simulink model "sim3_3"  (R2019a)
settings: Solver=VariableStepAuto  StartTime=0.0  StopTime=10.0  RelTol=1e-3
values from neighbouring files (symbols this model uses):
  h = 0.2    [matlab3_3.m]
  Ki_a = 25    [matlab3_3.m]
  Ki_d = Ki_a * h / 2    (= 2.5)    [matlab3_3.m]
  Kp_a = 6    [matlab3_3.m]
  Kp_d = Kp_a    (= 6)    [matlab3_3.m]
undefined symbols (not defined in the file or in its folder): denG, numG
settings Model: Creator=User  LastModifiedBy=User

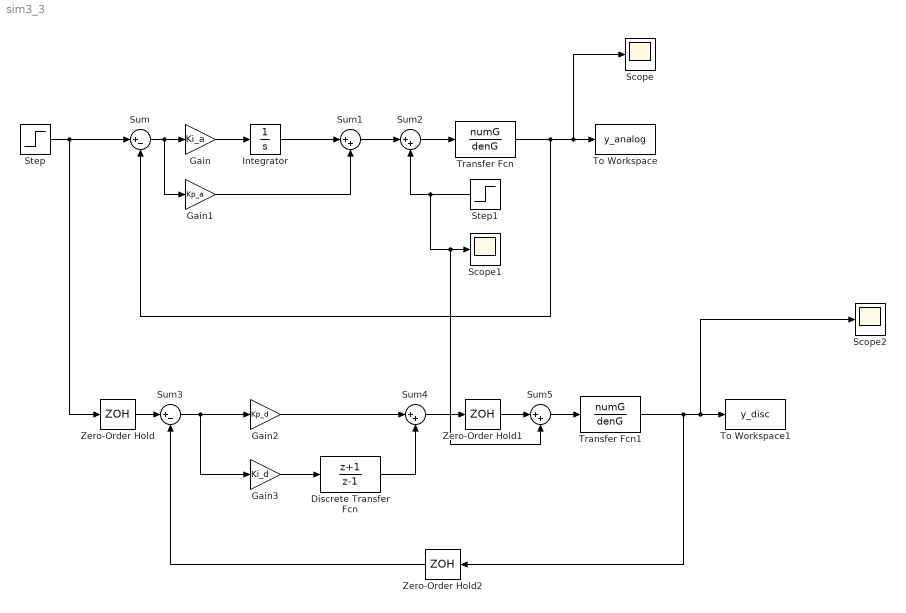
== system sim3_3 ==
  Discrete Transfer Fcn : DiscreteTransferFcn  Numerator=[1 1]  Denominator=[1 -1]  SampleTime=h
  Gain : Gain  Gain=Ki_a
  Gain1 : Gain  Gain=Kp_a
  Gain2 : Gain  Gain=Kp_d
  Gain3 : Gain  Gain=Ki_d
  Integrator : Integrator
  Scope : Scope
  Scope1 : Scope
  Scope2 : Scope
  Step : Step  SampleTime=0
  Step1 : Step  Time=0  After=0  SampleTime=0
  Sum : Sum  Inputs=|+-
  Sum{1..2,4..5} (4 alike) : Sum  Inputs=|++
  Sum3 : Sum  Inputs=|+-
  To Workspace : ToWorkspace  VariableName=y_analog  SaveFormat=Structure With Time  SampleTime=-1
  To Workspace1 : ToWorkspace  VariableName=y_disc  SaveFormat=Structure With Time  SampleTime=-1
  Transfer Fcn : TransferFcn  Numerator=numG  Denominator=denG
  Transfer Fcn1 : TransferFcn  Numerator=numG  Denominator=denG
  Zero-Order Hold : ZeroOrderHold  SampleTime=h
  Zero-Order Hold1 : ZeroOrderHold  SampleTime=h
  Zero-Order Hold2 : ZeroOrderHold  SampleTime=h
  wires:
  Sum/1 -> Gain1/1, Gain/1
  Gain/1 -> Integrator/1
  Integrator/1 -> Sum1/1
  Gain1/1 -> Sum1/2
  Sum2/1 -> Transfer Fcn/1
  Sum1/1 -> Sum2/1
  Transfer Fcn/1 -> Scope/1, To Workspace/1, Sum/2
  Step/1 -> Zero-Order Hold/1, Sum/1
  Sum3/1 -> Gain3/1, Gain2/1
  Gain2/1 -> Sum4/1
  Gain3/1 -> Discrete Transfer Fcn/1
  Discrete Transfer Fcn/1 -> Sum4/2
  Sum4/1 -> Zero-Order Hold1/1
  Step1/1 -> Sum5/2, Scope1/1, Sum2/2
  Sum5/1 -> Transfer Fcn1/1
  Transfer Fcn1/1 -> Scope2/1, To Workspace1/1, Zero-Order Hold2/1
  Zero-Order Hold/1 -> Sum3/1
  Zero-Order Hold1/1 -> Sum5/1
  Zero-Order Hold2/1 -> Sum3/2
